simulink subsystem "decYear2yearDOYsec"  (R2025b)
settings: Solver=VariableStepAuto  StartTime=0.0  StopTime=10.0  RelTol=1e-3
settings Model: Creator=antoniohernandez-rodiciomateos  LastModifiedBy=antoniohernandez-rodiciomateos

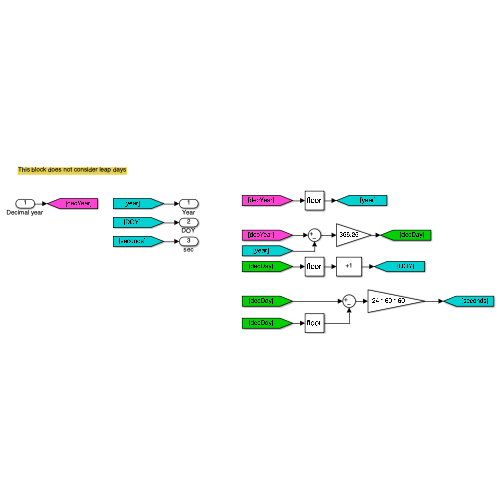
[thumbnail: Simulink's stored preview of the top-level diagram]
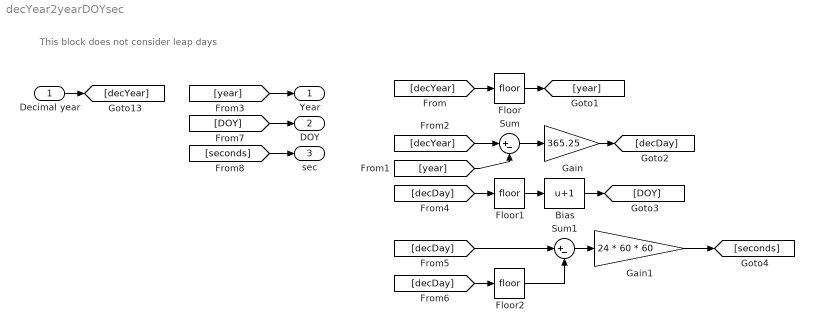
== system decYear2yearDOYsec ==
  note: This block does not consider leap days
  Decimal year : Inport  OutDataTypeStr=double  PortDimensions=[1 1]
  Bias : Bias  Bias=1  SaturateOnIntegerOverflow=off
  Floor : Rounding
  Floor1 : Rounding
  Floor2 : Rounding
  Gain : Gain  Gain=365.25
  Gain1 : Gain  Gain=24 * 60 * 60
  Sum : Sum  Inputs=|+-
  Sum1 : Sum  Inputs=|+-
  Year : Outport  OutDataTypeStr=double  PortDimensions=[1 1]
  DOY : Outport  Port=2  OutDataTypeStr=double  PortDimensions=[1 1]
  sec : Outport  Port=3  OutDataTypeStr=double  PortDimensions=[1 1]
  wires:
  Decimal year/1 -> [decYear]
  [decYear] -> Floor/1
  Floor/1 -> [year]
  [decYear] -> Sum/1
  [year] -> Sum/2
  [year] -> Year/1
  [decDay] -> Floor1/1
  Sum/1 -> Gain/1
  Gain/1 -> [decDay]
  Floor1/1 -> Bias/1
  Bias/1 -> [DOY]
  [decDay] -> Sum1/1
  [decDay] -> Floor2/1
  Floor2/1 -> Sum1/2
  Sum1/1 -> Gain1/1
  [DOY] -> DOY/1
  Gain1/1 -> [seconds]
  [seconds] -> sec/1
